simulink model "gm_uz_interlockDeadtime2L_vnl"  (R2020b)
settings: Solver=FixedStepDiscrete  StartTime=0.0  StopTime=0.01  RelTol=1e-3
libraries: simulink x17, hdlmdlgenlib x12, hdlsllib x7, eePwmGeneratorTwoLevel x1, powerlib_meascontrol x1
(part 2 of 2)

== system gm_uz_interlockDeadtime2L_vnl/uz_interlockDeadtime2L/InverseBotSwitchModule_instance1 ==
  gate_delay_out : Inport  OutDataTypeStr=boolean  PortDimensions=[2]  SampleTime=1e-08
  inverse_bottom_switch : Inport  Port=2  OutDataTypeStr=boolean  PortDimensions=1  SampleTime=1e-08
  Index Vector : MultiPortSwitch  DataPortOrder=Zero-based contiguous  Inputs=2  DiagnosticForDefault=None  zeroidx=on  SampleTime=1e-08
  NOT : Logic  Operator=NOT  Inputs=1  AllPortsSameDT=off  OutDataTypeStr=boolean  SampleTime=1e-08
  PipeDelay : Delay  DelayLength=double(1)  InitialCondition=0  SampleTime=1e-08
  gate_delay_out_0_wire : hdlmdlgenlib/Buffer
      settings: SourceProductBaseCode=SL
  gate_delay_out_1_wire : hdlmdlgenlib/Buffer
      settings: SourceProductBaseCode=SL
  mux : Mux  Inputs=2
  t : Demux  Outputs=2
  gate_enable_out : Outport
  wires:
  t/2 -> gate_delay_out_1_wire/1
  t/1 -> gate_delay_out_0_wire/1
  gate_delay_out_1_wire/1 -> NOT/1, Index Vector/2
  gate_delay_out_0_wire/1 -> mux/1
  Index Vector/1 -> mux/2
  mux/1 -> gate_enable_out/1
  NOT/1 -> Index Vector/3
  PipeDelay/1 -> Index Vector/1
  inverse_bottom_switch/1 -> PipeDelay/1
  gate_delay_out/1 -> t/1

== system gm_uz_interlockDeadtime2L_vnl/uz_interlockDeadtime2L/InverseBotSwitchModule_instance2 ==
  gate_delay_out : Inport  OutDataTypeStr=boolean  PortDimensions=[2]  SampleTime=1e-08
  inverse_bottom_switch : Inport  Port=2  OutDataTypeStr=boolean  PortDimensions=1  SampleTime=1e-08
  Index Vector : MultiPortSwitch  DataPortOrder=Zero-based contiguous  Inputs=2  DiagnosticForDefault=None  zeroidx=on  SampleTime=1e-08
  NOT : Logic  Operator=NOT  Inputs=1  AllPortsSameDT=off  OutDataTypeStr=boolean  SampleTime=1e-08
  PipeDelay : Delay  DelayLength=double(1)  InitialCondition=0  SampleTime=1e-08
  gate_delay_out_0_wire : hdlmdlgenlib/Buffer
      settings: SourceProductBaseCode=SL
  gate_delay_out_1_wire : hdlmdlgenlib/Buffer
      settings: SourceProductBaseCode=SL
  mux : Mux  Inputs=2
  t : Demux  Outputs=2
  gate_enable_out : Outport
  wires:
  gate_delay_out/1 -> t/1
  inverse_bottom_switch/1 -> PipeDelay/1
  PipeDelay/1 -> Index Vector/1
  NOT/1 -> Index Vector/3
  mux/1 -> gate_enable_out/1
  Index Vector/1 -> mux/2
  gate_delay_out_0_wire/1 -> mux/1
  gate_delay_out_1_wire/1 -> Index Vector/2, NOT/1
  t/1 -> gate_delay_out_0_wire/1
  t/2 -> gate_delay_out_1_wire/1

== system gm_uz_interlockDeadtime2L_vnl/uz_interlockDeadtime2L/InverseBotSwitchModule_instance3 ==
  gate_delay_out : Inport  OutDataTypeStr=boolean  PortDimensions=[2]  SampleTime=1e-08
  inverse_bottom_switch : Inport  Port=2  OutDataTypeStr=boolean  PortDimensions=1  SampleTime=1e-08
  Index Vector : MultiPortSwitch  DataPortOrder=Zero-based contiguous  Inputs=2  DiagnosticForDefault=None  zeroidx=on  SampleTime=1e-08
  NOT : Logic  Operator=NOT  Inputs=1  AllPortsSameDT=off  OutDataTypeStr=boolean  SampleTime=1e-08
  PipeDelay : Delay  DelayLength=double(1)  InitialCondition=0  SampleTime=1e-08
  gate_delay_out_0_wire : hdlmdlgenlib/Buffer
      settings: SourceProductBaseCode=SL
  gate_delay_out_1_wire : hdlmdlgenlib/Buffer
      settings: SourceProductBaseCode=SL
  mux : Mux  Inputs=2
  t : Demux  Outputs=2
  gate_enable_out : Outport
  wires:
  gate_delay_out/1 -> t/1
  inverse_bottom_switch/1 -> PipeDelay/1
  PipeDelay/1 -> Index Vector/1
  NOT/1 -> Index Vector/3
  mux/1 -> gate_enable_out/1
  Index Vector/1 -> mux/2
  gate_delay_out_0_wire/1 -> mux/1
  gate_delay_out_1_wire/1 -> Index Vector/2, NOT/1
  t/1 -> gate_delay_out_0_wire/1
  t/2 -> gate_delay_out_1_wire/1

== system gm_uz_interlockDeadtime2L_vnl/uz_interlockDeadtime2L_vnl/DeadtimeModule ==
  note: This delay is only used to improve timing (Pipeline) and is not related to the function of the module!
  note: Resets the counter at a falling edge
  In1 : Inport  Partition=on  PartitionDimension=1  PartitionWidth=1  PartitionOffset=0
  DelayCycles : Inport  Port=2
  Delay2 : Delay  DelayLength=1  ExternalReset=Level
      settings: InputPortMap=u0,r5
  Detect Fall Nonpositive2 : simulink/Logic and Bit Operations/Detect Fall Nonpositive  vinit=0  OutDataTypeStr=boolean
      settings: SourceProductBaseCode=SL
  For Each : ForEach  DisableCoverage=on
  HDL Counter : hdlsllib/Sources/HDL Counter  CountType=Free running  CountInit=0  CountStep=1  CountMax=25  CountFromType=Initial value  CountFrom=0  CountResetPort=on  CountLoadPort=off  CountEnbPort=on  CountDirPort=off  CountDataType=Unsigned  CountWordLen=10  CountFracLen=0  CountSampTime=-1
  Logical Operator10 : Logic  AllPortsSameDT=off  OutDataTypeStr=boolean
  PipelineDelay1 : Delay  DelayLength=1
  Relational Operator : RelationalOperator  Operator===  OutDataTypeStr=boolean  RndMeth=Simplest
  Switch : Switch  Criteria=u2 ~= 0  Threshold=1
  gate_delay_out : Outport  ConcatenationDimension=1
  wires:
  Logical Operator10/1 -> gate_delay_out/1
  Switch/1 -> Logical Operator10/2, Delay2/1
  PipelineDelay1/1 -> Delay2/2, HDL Counter/1
  Relational Operator/1 -> Switch/2
  Detect Fall Nonpositive2/1 -> PipelineDelay1/1
  HDL Counter/1 -> Relational Operator/2
  Delay2/1 -> Switch/3
  DelayCycles/1 -> Relational Operator/1
  In1/1 -> Detect Fall Nonpositive2/1, HDL Counter/2, Switch/1, Logical Operator10/1

== system gm_uz_interlockDeadtime2L_vnl/uz_interlockDeadtime2L_vnl/EnableOutputModule ==
  gate_delay_out : Inport  Partition=on  PartitionDimension=1  PartitionWidth=1  PartitionOffset=0
  enable : Inport  Port=2
  AND : Logic  AllPortsSameDT=off  OutDataTypeStr=boolean
  For Each : ForEach  DisableCoverage=on
  gate_enable_out : Outport  ConcatenationDimension=1
  wires:
  AND/1 -> gate_enable_out/1
  gate_delay_out/1 -> AND/1
  enable/1 -> AND/2

== system gm_uz_interlockDeadtime2L_vnl/uz_interlockDeadtime2L_vnl/InterlockModule ==
  In1 : Inport  Partition=on  PartitionDimension=1  PartitionWidth=2  PartitionOffset=0
  Demux : Demux  Outputs=2
  For Each : ForEach  DisableCoverage=on
  Logical Operator1 : Logic  AllPortsSameDT=off  OutDataTypeStr=boolean
  Logical Operator2 : Logic  AllPortsSameDT=off  OutDataTypeStr=boolean
  Logical Operator3 : Logic  Operator=NOT  AllPortsSameDT=off  OutDataTypeStr=boolean
  Logical Operator4 : Logic  Operator=NOT  AllPortsSameDT=off  OutDataTypeStr=boolean
  Mux : Mux  Inputs=2
  gate_delay_out : Outport  ConcatenationDimension=1
  wires:
  In1/1 -> Demux/1
  Mux/1 -> gate_delay_out/1
  Logical Operator4/1 -> Logical Operator1/1
  Logical Operator2/1 -> Mux/1  "PWM_AH"
  Logical Operator3/1 -> Logical Operator2/2
  Demux/2 -> Logical Operator3/1, Logical Operator1/2
  Logical Operator1/1 -> Mux/2  "interlock_bot_out"
  Demux/1 -> Logical Operator2/1, Logical Operator4/1

== system gm_uz_interlockDeadtime2L_vnl/uz_interlockDeadtime2L_vnl/InverseBotSwitchModule ==
  gate_delay_out : Inport  Partition=on  PartitionDimension=1  PartitionWidth=2  PartitionOffset=0
  inverse_bottom_switch : Inport  Port=2
  Demux : Demux  Outputs=2
  For Each : ForEach  DisableCoverage=on
  Index Vector : MultiPortSwitch  DataPortOrder=Zero-based contiguous  Inputs=2  zeroidx=on
  Mux : Mux  Inputs=2
  NOT : Logic  Operator=NOT  AllPortsSameDT=off  OutDataTypeStr=boolean
  PipeDelay : Delay  DelayLength=1
  gate_enable_out : Outport  ConcatenationDimension=1
  wires:
  gate_delay_out/1 -> Demux/1
  Mux/1 -> gate_enable_out/1
  NOT/1 -> Index Vector/3
  Demux/1 -> Mux/1
  inverse_bottom_switch/1 -> PipeDelay/1
  Index Vector/1 -> Mux/2
  Demux/2 -> NOT/1, Index Vector/2
  PipeDelay/1 -> Index Vector/1
